simulink model "prakt5"  (R2025b)
settings: Solver=VariableStepAuto  StartTime=0.0  StopTime=10.0  RelTol=1e-3
settings Model: Creator=danieltchoudovski  LastModifiedBy=danieltchoudovski

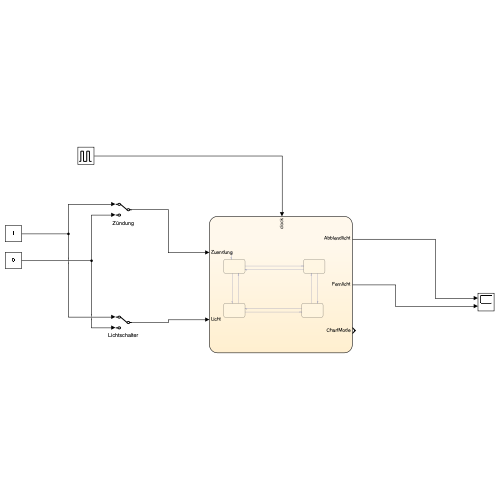
[thumbnail: Simulink's stored preview of the top-level diagram]
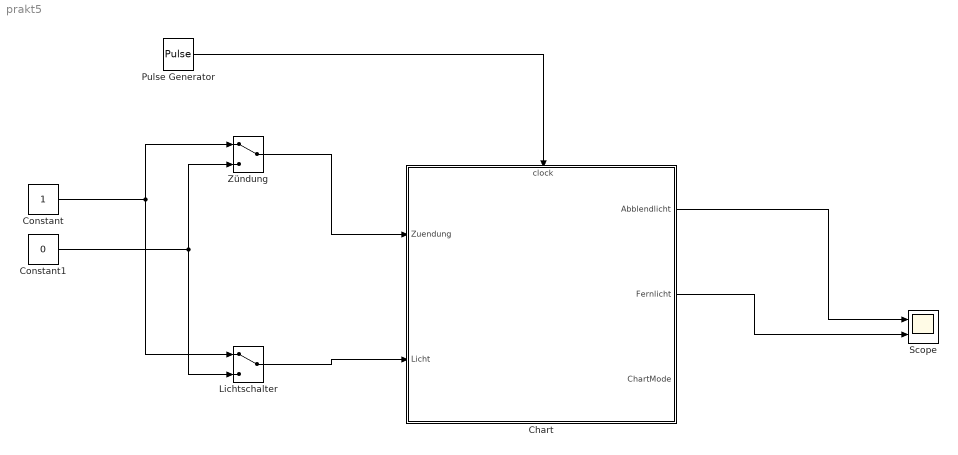
== system prakt5 ==
  Chart : Stateflow chart  TreatAsAtomicUnit=on
      settings: PortSchema="{\"entries\":[{\"content\":{\"sides\":[{\"content\":{\"connectorIds\":[\"In2\",\"In3\"]},\"type\":\"ConnectorPlacement.EquallySpacedRectSide\",\"uuid\":\"c64f2c48-f71d-4338-90cb-3285749ff8d0\"},{\"content\":{\"connectorIds\":[\"Out1\",\"Out2\",\"Out3\"],\"side\":\"RIGHT\"},\"type\":\"ConnectorPlacement.EquallySpacedRectSide\",\"uuid\":\"da078766-d03f-4257-8d31-e5009b8c0c51\"},{\"content\":{\"connectorIds\":[\"In1\"],\"side\":\"TOP\"},\"type\":\"ConnectorPlacement.EquallySpacedRectSide\",\"uuid\":\"252c41eb-6376-41bb-a58a-4166c84b9a80\"}]},\"type\":\"ConnectorPlacement.EquallySpacedConnector\",\"uuid\":\"4a56fa51-ba47-40c2-b670-d54020af6d09\"}],\"packageUris\":[\"http://schema.mathworks.com/mf0/Connector/R2020b\"],\"version\":\"1.0\"}"
  Constant : Constant
  Constant1 : Constant  Value=0
  Lichtschalter : ManualSwitch
  Pulse Generator : DiscretePulseGenerator  PulseType=Time based  Period=0.1  PulseWidth=5
  Scope : Scope  NumInputPorts=2
      settings: ActiveDisplayYMinimum=-0.12499999999999997  ActiveDisplayYMaximum=1.125
  Zündung : ManualSwitch
  wires:
  Constant/1 -> Lichtschalter/1, Zündung/1
  Constant1/1 -> Zündung/2, Lichtschalter/2
  Zündung/1 -> Chart/2(Zuendung)
  Lichtschalter/1 -> Chart/3(Licht)
  Pulse Generator/1 -> Chart/1(clock)
  Chart/1(Abblendlicht) -> Scope/1
  Chart/2(Fernlicht) -> Scope/2

== stateflow chart prakt5/Chart ==
  settings: executeAtInitialization=1
  state Z0L0
    en:
    Abblendlicht = 0;
    Fernlicht = 0;
  state Z1L0
    en:
    Abblendlicht = 1;
    Fernlicht = 0;
  state Z0L1
    en:
    Abblendlicht = 1;
    Fernlicht = 0;
  state Z1L1
    en:
    Abblendlicht = 0;
    Fernlicht = 1;
  (default) -> Z0L0
  Z0L0 -> Z1L0 [order 1] : [Zuendung == 1]
  Z1L0 -> Z0L0 [order 2] : [Zuendung == 0]
  Z0L0 -> Z0L1 [order 2] : [Licht ==1]
  Z0L1 -> Z0L0 [order 2] : [Licht == 0]
  Z1L1 -> Z1L0 [order 1] : [Licht == 0]
  Z1L0 -> Z1L1 [order 1] : [Licht == 1]
  Z1L1 -> Z0L1 [order 2] : [Zuendung == 0]
  Z0L1 -> Z1L1 [order 1] : [Zuendung ==1]
  data: clock input; Zuendung input; Licht input; Abblendlicht output; Fernlicht output; ChartMode output Enum: ChartModeType
